simulink model "Whisper"  (R2020a)
settings: Solver=VariableStepAuto  StartTime=0.0  StopTime=Inf  RelTol=1e-3
libraries: dspxfrm3 x3, dspsigops x2, dspsnks4 x1, dspvision x1, dspsrcs4 x1
settings Model: Creator=miche  LastModifiedBy=miche

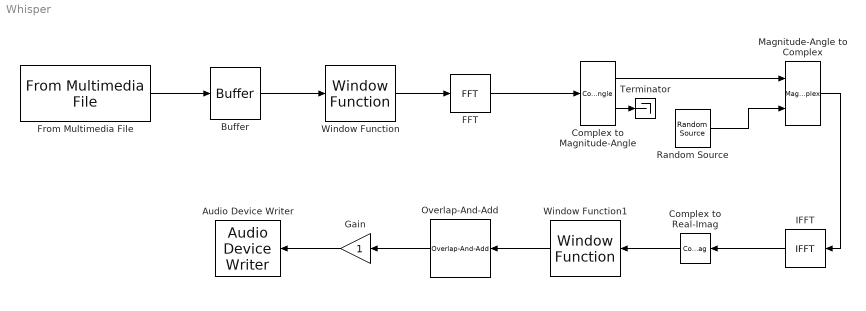
== system Whisper ==
  Audio Device Writer : dspsnks4/Audio Device Writer  Driver=DirectSound  Device=Default  InheritSampleRate=on  SampleRate=44100  BitDepth=16-bit integer  BufferSize=4096  NumBuffers=10  DefaultOutputChannelMapping=on  OutputChannelMapping=1:2  OutputNumUnderrunSamples=off  DriverIdx=1  DeviceWarnFlag=''
  Buffer : Buffer  N=1024  V=960  OutputFrames=off
  Complex to Magnitude-Angle : ComplexToMagnitudeAngle
  Complex to Real-Imag : ComplexToRealImag  Output=Real
  FFT : dspxfrm3/FFT  FFTImplementation=Auto  CompMethod=Table lookup  TableOpt=NEW  TableOptActive=Speed  BitRevOrder=off  Normalize=off  InheritFFTLength=on  FFTLength=64  WrapInput=on  roundingMode=Floor  overflowMode=off  firstCoeffDataTypeStr=Inherit: Same word length as input  firstCoeffLastDataTypeStr=Inherit: Same word length as input  outputMin=[]  outputMax=[]
  From Multimedia File : dspvision/From Multimedia File  inputFilename=C:\Users\miche\Documents\MATLAB\audio.wav  readRange=[1 Inf]  loop=on  numPlays=inf  outputStreams=Audio only  videoDataType=single  audioDataType=double  inheritSampleTime=on  userDefinedSampleTime=1/30  noAudioOutput=off  isIntensityVideo=off  fourcc=RGB  colorVideoFormat=Separate color signals  outputEOF=off  dataOrg=Column-major  audioFrameSize=1024  computeAudioFrameSize=off  outSamplingMode=Sample based
  Gain : Gain
  IFFT : dspxfrm3/IFFT  FFTImplementation=Auto  CompMethod=Table lookup  TableOpt=NEW  TableOptActive=Speed  BitRevOrder=off  cs_in=off  Normalize=on  InheritFFTLength=on  FFTLength=64  WrapInput=on  mode=Complex  outSamplingMode=Sample based  roundingMode=Floor  overflowMode=off  firstCoeffDataTypeStr=Inherit: Same word length as input  firstCoeffLastDataTypeStr=Inherit: Same word length as input  outputMin=[]  outputMax=[]
  Magnitude-Angle to Complex : MagnitudeAngleToComplex
  Overlap-And-Add : dspxfrm3/Inverse  Short-Time FFT/Overlap-And-Add  L=64
      settings: SourceProductBaseCode=DS
  Random Source : dspsrcs4/Random Source  SrcType=Uniform  NormMethod=Ziggurat  CltLength=12  MinVal=0  MaxVal=2*pi  MeanVal=0  VarVal=1  RepMode=Not repeatable  rawSeed=1  IsInherit=on  SampMode=Discrete  SampTime=1  SampFrame=1024  DataType=Double  OutComplex=Real  OutputFrames=off
  Terminator : Terminator
  Window Function : dspsigops/Window Function  winmode=Apply window to input  wintype=Hanning  sampmode=Continuous  samptime=1  N=1024  Rs=50  beta=10  winsamp=Periodic  UserWindow=hamming  OptParams=off  UserParams={'symmetric'}  dataType=double  isSigned=on  wordLen=16  udDataType=sfix(16)  fracBitsMode=Best precision  numFracBits=15  roundingMode=Floor  overflowMode=off  numSidelobes=4  sidelobeLevel=-30
      settings: SourceProductBaseCode=DS
  Window Function1 : dspsigops/Window Function  winmode=Apply window to input  wintype=Hanning  sampmode=Continuous  samptime=1  N=1024  Rs=50  beta=10  winsamp=Periodic  UserWindow=hamming  OptParams=off  UserParams={'symmetric'}  dataType=double  isSigned=on  wordLen=16  udDataType=sfix(16)  fracBitsMode=Best precision  numFracBits=15  roundingMode=Floor  overflowMode=off  numSidelobes=4  sidelobeLevel=-30
      settings: SourceProductBaseCode=DS
  wires:
  Gain/1 -> Audio Device Writer/1
  Overlap-And-Add/1 -> Gain/1
  Buffer/1 -> Window Function/1
  FFT/1 -> Complex to Magnitude-Angle/1
  IFFT/1 -> Complex to Real-Imag/1
  Window Function/1 -> FFT/1
  Complex to Real-Imag/1 -> Window Function1/1
  Complex to Magnitude-Angle/2 -> Terminator/1
  Random Source/1 -> Magnitude-Angle to Complex/2
  Magnitude-Angle to Complex/1 -> IFFT/1
  From Multimedia File/1 -> Buffer/1
  Window Function1/1 -> Overlap-And-Add/1
  Complex to Magnitude-Angle/1 -> Magnitude-Angle to Complex/1
